simulink library "CElib"  (R2021a)
settings: Solver=VariableStepAuto  StartTime=0.0  StopTime=10.0  RelTol=1e-3
settings Model: Creator=MSI-NB  LastModifiedBy=MSI-NB

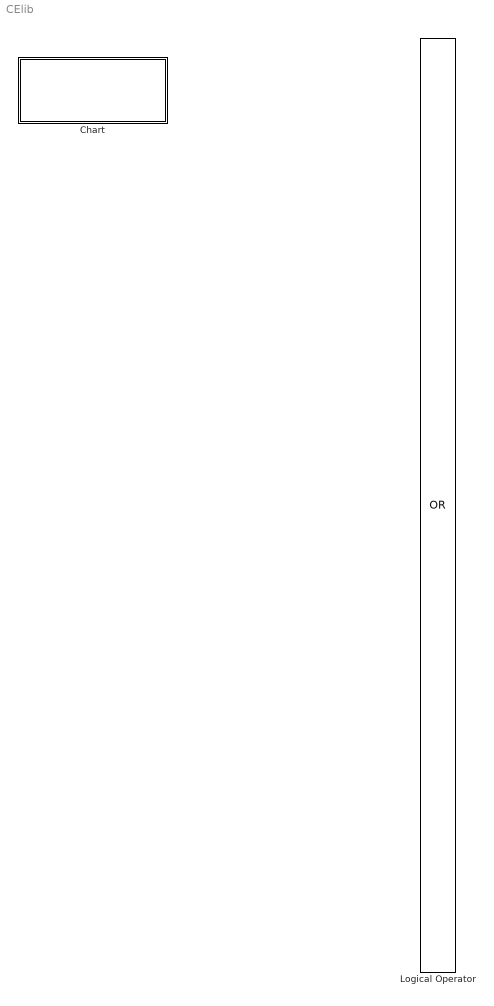
== system CElib ==
  Chart : Stateflow chart  TreatAsAtomicUnit=on
  Logical Operator : Logic  Operator=OR  Inputs=9  AllPortsSameDT=off  OutDataTypeStr=boolean

== stateflow chart CElib/Chart ==
  state off
  state on
    state initial
    state CE2
    state CE3
    state CE1
    (default) -> initial
    (junction 21) -> initial
    (junction 27) -> initial
    CE2 -> (junction 21) [order 2]
    CE1 -> (junction 27) [order 2]
    initial -> (junction 28) [order 3]
    initial -> (junction 23) [order 2]
    (junction 28) -> CE1
    (junction 23) -> CE2
    initial -> CE3 [order 1]
    CE3 -> initial [order 1]
    CE2 -> CE3 [order 1]
    CE3 -> CE1 [order 2]
    CE1 -> CE3 [order 1]
    CE3 -> CE2 [order 3]
    CE2 -> (junction 36) [order 3]
    (junction 33) -> CE2
    CE1 -> (junction 39) [order 3]
    (junction 38) -> CE1
    (junction 39) -> (junction 33)
    (junction 36) -> (junction 38)
  (default) -> off
  off -> on
  on -> off
